simulink model "MP_BearinglessMotor"  (R2024b)
settings: Solver=FixedStepAuto  StartTime=0  StopTime=Tend  FixedStep=Tsim  RelTol=1e-3
values from neighbouring files (symbols this model uses):
  alpha_s = 2*pi/m*ps    (= 5.23598775598)    [setup.m]
  alpha_t = 2*pi/m*p    (= 4.18879020479)    [setup.m]
  Fx_hat = 2/m*Kf    (= 0.6)    [setup.m]
  Fy_hat = 2/m*Kf    (= 0.6)    [setup.m]
  Ke = 0.003    [setup.m]
  p = 4    [setup.m]
  tau_hat = 2/m*Kt    (= 0.00666666666667)    [setup.m]
  Tsim = 1e-8    (= 1e-08)    [setup.m]
  V_DC = 160    [setup.m]
libraries: spsControlledVoltageSourceLib x12, spsIdealSwitchLib x12, spsCurrentMeasurementLib x6, spsMutualInductanceLib x1, spsTriangleGeneratorLib x1, spsVoltageMeasurementLib x1, spsDCVoltageSourceLib x1, spspowerguiLib x1
settings Model: Creator=chiba  LastModifiedBy=tnoguchi
settings SolverCC: AllowMultiTaskInputOutput=on
settings DataIOCC: SaveOutput=off  SaveTime=off
settings OptimizationCC: DefaultParameterBehavior=Inlined  ReuseModelBlockBuffer=off  EnhancedBackFolding=on  PassReuseOutputArgsAs=Individual arguments  ZeroExternalMemoryAtStartup=off  ZeroInternalMemoryAtStartup=off  OptimizeBlockOrder=speed  DifferentSizesBufferReuse=on  EfficientTunableParamExpr=on
settings DebuggingCC: ParameterTunabilityLossMsg=error
settings SFSimCC: MATLABDynamicMemAlloc=off
settings RTWCC: Description=Embedded Coder  SystemTargetFile=ert.tlc  TemplateMakefile=ert_default_tmf  GPUComputeCapability=3.5
settings CodeAppCC: ForceParamTrailComments=on  IgnoreCustomStorageClasses=off  OperatorAnnotations=on  SimulinkDataObjDesc=on  SFDataObjDesc=on  InsertBlockDesc=on
settings ERTTargetCC: TargetLangStandard=C99 (ISO)  ERTCustomFileTemplate=example_file_process.tlc  DynamicArrayContainerType=coder::array

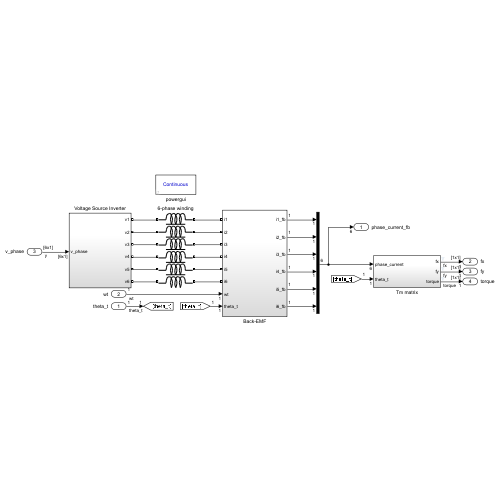
[thumbnail: Simulink's stored preview of the top-level diagram]
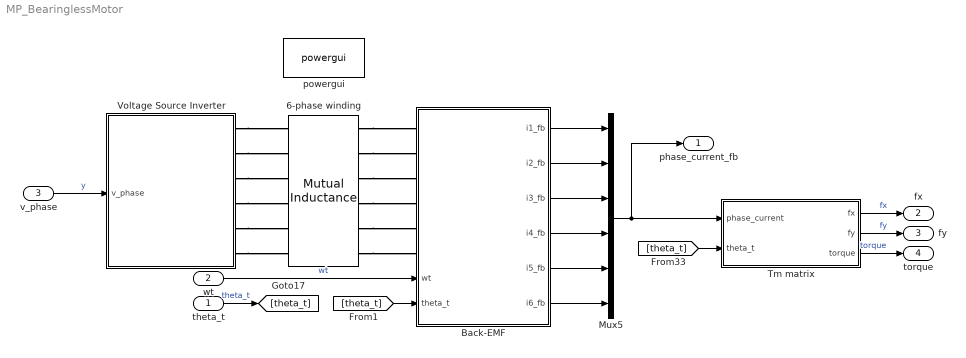
== system MP_BearinglessMotor ==
  theta_t : Inport  OutDataTypeStr=double  PortDimensions=1  SampleTime=0
  wt : Inport  Port=2  OutDataTypeStr=double  PortDimensions=1
  v_phase : Inport  Port=3  OutDataTypeStr=double  PortDimensions=[6 1]  SampleTime=0
  6-phase winding : spsMutualInductanceLib/Mutual Inductance  LConnTagsString=a|b|c|L4|L5|L6  RConnTagsString=A|B|C|R4|R5|R6  TypeOfMutual=Generalized mutual inductance  NumberOfWindings=6  SelfImpedance1=[1.1 1.1e-03]  SelfImpedance2=[ 1.1 1.1e-03]  ThreeWindings=on  SelfImpedance3=[ 1.1 1.1e-03]  MutualImpedance=[1.0 1.0e-03]  InductanceMatrix=Lmat  ResistanceMatrix=Rmat  Measurements=None
      settings: LibrarySourceBlock=sps_lib/Passives/Mutual Inductance
  Back-EMF : Subsystem
      settings: PortSchema="{\"entries\":[{\"content\":{\"sides\":[{\"content\":{\"connectorIds\":[\"LConn1\",\"LConn2\",\"LConn3\",\"LConn4\",\"LConn5\",\"LConn6\",\"In1\",\"In2\"]},\"type\":\"ConnectorPlacement.EquallySpacedRectSide\",\"uuid\":\"749577e6-e43c-48b0-9a92-cb274024c2f1\"},{\"content\":{\"connectorIds\":[\"Out1\",\"Out2\",\"Out3\",\"Out4\",\"Out5\",\"Out6\"],\"side\":\"RIGHT\"},\"type\":\"ConnectorPlacement.EquallySpacedRectSide\",\"uuid\":\"b47f9487-f754-4b9c-a86a-8672228b8979\"},{\"content\":{\"side\":\"TOP\"},\"type\":\"ConnectorPlacement.EquallySpacedRectSide\",\"uuid\":\"ca9d39d3-2f68-4271-a0d3-29a08329b066\"}]},\"type\":\"ConnectorPlacement.EquallySpacedConnector\",\"uuid\":\"24c892f7-b8cb-4be8-a5cc-492343e32fdb\"}],\"packageUris\":[\"http://schema.mathworks.com/mf0/Connector/R2020b\"],\"version\":\"1.0\"}"
  Mux5 : Mux  Inputs=6
  Tm matrix : Subsystem
  Voltage Source Inverter : Subsystem
  powergui : spspowerguiLib/powergui  Priority=1  SimulationMode=Continuous  SampleTime=Tsim  frequency=60  Iterations=50  frequencyindice=0  Pbase=100e6  ErrMax=1e-4  UnitsV=kV  UnitsW=MW  buscounter=0  FunctionMessages=off  echomessages=off  EnableUseOfTLC=off  CurrentSourceSwitches=off  DisableSnubberDevices=off  DisableRonSwitches=off  DisableVfSwitches=off  DisplayEquations=off  AutomaticDiscreteSolvers=off  SolverType=Tustin/Backward Euler (TBE)  Interpol=off  ExternalGateDelay=off  methode=off  Ts=100  x0status=blocks  SPID=on  SwTol=0  HookPort=off  NonlinearTolerance=1e-4  nMaxIteration=100  ContinueOnMaxIteration=off  RestoreLinks=warning  ResistiveCurrentMeasurement=off  Frange=[0:2:500]  Ylog=off  Xlog=on  ShowGrid=off  save=off  variable=ZData  structure=0  ZoomFFT=off  StartTime=0.0  cycles=1  DisplayStyle=1  fundamental=60  FreqAxis=off  MaxFrequency=1000  frequencyindicesteady=1  RmsSteady=1  display=off
  phase_current_fb : Outport  OutDataTypeStr=double  PortDimensions=6  SampleTime=0
  fx : Outport  Port=2  OutDataTypeStr=double  PortDimensions=1  SampleTime=0
  fy : Outport  Port=3  OutDataTypeStr=double  PortDimensions=1  SampleTime=0
  torque : Outport  Port=4  OutDataTypeStr=double  PortDimensions=1  SampleTime=0
  wires:
  Back-EMF/1(i1_fb) -> Mux5/1
  Back-EMF/3(i3_fb) -> Mux5/3
  Back-EMF/2(i2_fb) -> Mux5/2
  Back-EMF/5(i5_fb) -> Mux5/5
  Back-EMF/4(i4_fb) -> Mux5/4
  Back-EMF/6(i6_fb) -> Mux5/6
  [theta_t] -> Tm matrix/2(theta_t)
  Mux5/1 -> Tm matrix/1(phase_current), phase_current_fb/1
  wt/1 -> Back-EMF/1(wt)  "wt"
  [theta_t] -> Back-EMF/2(theta_t)
  theta_t/1 -> [theta_t]  "theta_t"
  v_phase/1 -> Voltage Source Inverter/1(v_phase)  "y"
  Tm matrix/1(fx) -> fx/1  "fx"
  Tm matrix/2(fy) -> fy/1  "fy"
  Tm matrix/3(torque) -> torque/1  "torque"
  connections:
  6-phase winding/RConn1 -- Back-EMF/LConn1
  6-phase winding/RConn2 -- Back-EMF/LConn2
  6-phase winding/RConn3 -- Back-EMF/LConn3
  6-phase winding/RConn4 -- Back-EMF/LConn4
  6-phase winding/RConn5 -- Back-EMF/LConn5
  6-phase winding/RConn6 -- Back-EMF/LConn6
  Voltage Source Inverter/RConn5 -- 6-phase winding/LConn5
  Voltage Source Inverter/RConn6 -- 6-phase winding/LConn6
  Voltage Source Inverter/RConn4 -- 6-phase winding/LConn4
  Voltage Source Inverter/RConn3 -- 6-phase winding/LConn3
  Voltage Source Inverter/RConn2 -- 6-phase winding/LConn2
  Voltage Source Inverter/RConn1 -- 6-phase winding/LConn1

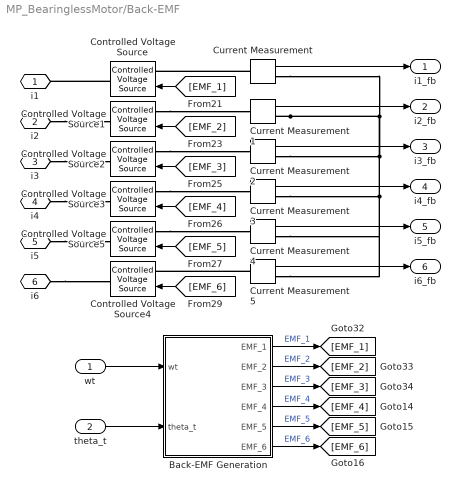
== system MP_BearinglessMotor/Back-EMF ==
  wt : Inport
  theta_t : Inport  Port=2
  Back-EMF Generation : Subsystem
  Controlled Voltage Source{,1..5} (6 alike) : spsControlledVoltageSourceLib/Controlled Voltage Source  Initialize=on  Source_Type=AC  Amplitude=0  Phase=0  Frequency=0  Measurements=None
  Current Measurement{,1..5} (6 alike) : spsCurrentMeasurementLib/Current Measurement  PhasorSimulation=off  OutputType=Complex  PSBequivalent=0
  i1 : PMIOPort  Side=Left
  i2 : PMIOPort  Port=2  Side=Left
  i3 : PMIOPort  Port=3  Side=Left
  i4 : PMIOPort  Port=4  Side=Left
  i5 : PMIOPort  Port=5  Side=Left
  i6 : PMIOPort  Port=6  Side=Left
  i1_fb : Outport
  i2_fb : Outport  Port=2
  i3_fb : Outport  Port=3
  i4_fb : Outport  Port=4
  i5_fb : Outport  Port=5
  i6_fb : Outport  Port=6
  wires:
  Current Measurement2/1 -> i3_fb/1
  Current Measurement4/1 -> i5_fb/1
  Back-EMF Generation/6(EMF_6) -> [EMF_6]  "EMF_6"
  [EMF_4] -> Controlled Voltage Source3/1
  Current Measurement1/1 -> i2_fb/1
  Back-EMF Generation/5(EMF_5) -> [EMF_5]  "EMF_5"
  Current Measurement3/1 -> i4_fb/1
  Back-EMF Generation/2(EMF_2) -> [EMF_2]  "EMF_2"
  [EMF_2] -> Controlled Voltage Source1/1
  [EMF_3] -> Controlled Voltage Source2/1
  [EMF_1] -> Controlled Voltage Source/1
  Current Measurement/1 -> i1_fb/1
  Back-EMF Generation/3(EMF_3) -> [EMF_3]  "EMF_3"
  Back-EMF Generation/4(EMF_4) -> [EMF_4]  "EMF_4"
  [EMF_6] -> Controlled Voltage Source4/1
  Back-EMF Generation/1(EMF_1) -> [EMF_1]  "EMF_1"
  wt/1 -> Back-EMF Generation/1(wt)
  [EMF_5] -> Controlled Voltage Source5/1
  theta_t/1 -> Back-EMF Generation/2(theta_t)
  Current Measurement5/1 -> i6_fb/1
  connections:
  i5/RConn1 -- Controlled Voltage Source5/RConn1
  i3/RConn1 -- Controlled Voltage Source2/RConn1
  Controlled Voltage Source2/LConn1 -- Current Measurement2/LConn1
  i6/RConn1 -- Controlled Voltage Source4/RConn1
  i4/RConn1 -- Controlled Voltage Source3/RConn1
  Controlled Voltage Source1/LConn1 -- Current Measurement1/LConn1
  Current Measurement1/RConn1 -- Current Measurement3/RConn1 -- Current Measurement5/RConn1 -- Current Measurement4/RConn1 -- Current Measurement2/RConn1 -- Current Measurement/RConn1
  Controlled Voltage Source/RConn1 -- i1/RConn1
  Current Measurement/LConn1 -- Controlled Voltage Source/LConn1
  Controlled Voltage Source3/LConn1 -- Current Measurement3/LConn1
  i2/RConn1 -- Controlled Voltage Source1/RConn1
  Controlled Voltage Source5/LConn1 -- Current Measurement4/LConn1
  Current Measurement5/LConn1 -- Controlled Voltage Source4/LConn1

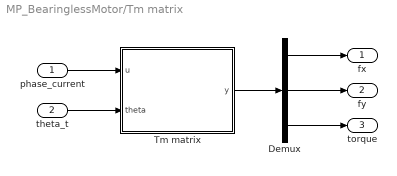
== system MP_BearinglessMotor/Tm matrix ==
  phase_current : Inport
  theta_t : Inport  Port=2
  Demux : Demux  Outputs=3
  Tm matrix : MATLAB Function  TreatAsAtomicUnit=on
  fx : Outport
  fy : Outport  Port=2
  torque : Outport  Port=3
  wires:
  phase_current/1 -> Tm matrix/1(u)
  Tm matrix/1(y) -> Demux/1
  Demux/1 -> fx/1
  Demux/2 -> fy/1
  Demux/3 -> torque/1
  theta_t/1 -> Tm matrix/2(theta)

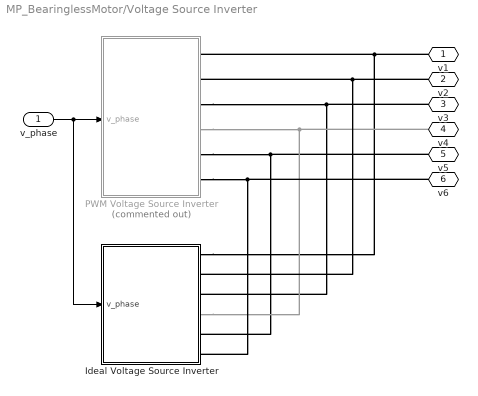
== system MP_BearinglessMotor/Voltage Source Inverter ==
  v_phase : Inport
  Ideal Voltage Source Inverter : Subsystem
  PWM Voltage Source Inverter : Subsystem  Commented=on
  v1 : PMIOPort  Side=Right
  v2 : PMIOPort  Port=2  Side=Right
  v3 : PMIOPort  Port=3  Side=Right
  v4 : PMIOPort  Port=4  Side=Right
  v5 : PMIOPort  Port=5  Side=Right
  v6 : PMIOPort  Port=6  Side=Right
  wires:
  v_phase/1 -> PWM Voltage Source Inverter/1(v_phase), Ideal Voltage Source Inverter/1(v_phase)
  connections:
  Ideal Voltage Source Inverter/RConn5 -- v5/RConn1 -- PWM Voltage Source Inverter/RConn5
  Ideal Voltage Source Inverter/RConn3 -- v3/RConn1 -- PWM Voltage Source Inverter/RConn3
  PWM Voltage Source Inverter/RConn1 -- v1/RConn1 -- Ideal Voltage Source Inverter/RConn1
  PWM Voltage Source Inverter/RConn4 -- v4/RConn1 -- Ideal Voltage Source Inverter/RConn4
  Ideal Voltage Source Inverter/RConn6 -- v6/RConn1 -- PWM Voltage Source Inverter/RConn6
  Ideal Voltage Source Inverter/RConn2 -- v2/RConn1 -- PWM Voltage Source Inverter/RConn2

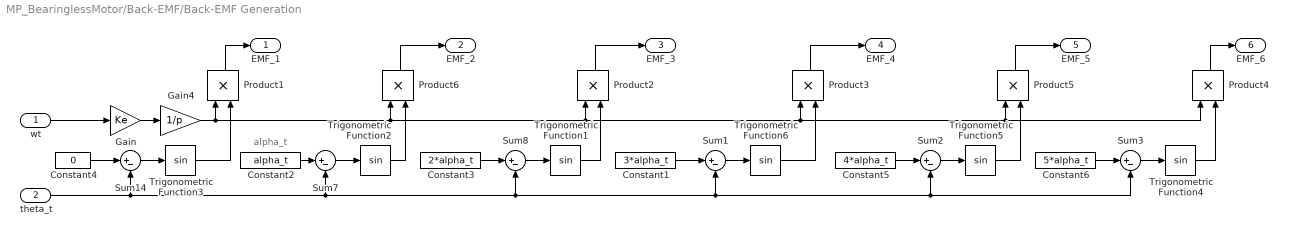
== system MP_BearinglessMotor/Back-EMF/Back-EMF Generation ==
  note: alpha_t
  wt : Inport
  theta_t : Inport  Port=2
  Constant1 : Constant  Value=3*alpha_t
  Constant2 : Constant  Value=alpha_t
  Constant3 : Constant  Value=2*alpha_t
  Constant4 : Constant  Value=0
  Constant5 : Constant  Value=4*alpha_t
  Constant6 : Constant  Value=5*alpha_t
  Gain : Gain  Gain=Ke
  Gain4 : Gain  Gain=1/p
  Product{1..6} (6 alike) : Product
  Sum{1..3,7..8,14} (6 alike) : Sum  Inputs=|+-
  Trigonometric Function{1..6} (6 alike) : Trigonometry
  EMF_1 : Outport
  EMF_2 : Outport  Port=2
  EMF_3 : Outport  Port=3
  EMF_4 : Outport  Port=4
  EMF_5 : Outport  Port=5
  EMF_6 : Outport  Port=6
  wires:
  Constant3/1 -> Sum8/1
  Product3/1 -> EMF_4/1
  Product5/1 -> EMF_5/1
  Product4/1 -> EMF_6/1
  Gain4/1 -> Product6/1, Product2/1, Product5/1, Product4/1, Product3/1, Product1/1
  Sum2/1 -> Trigonometric Function5/1
  Constant1/1 -> Sum1/1
  Constant5/1 -> Sum2/1
  Trigonometric Function5/1 -> Product5/2
  Constant6/1 -> Sum3/1
  Sum1/1 -> Trigonometric Function6/1
  theta_t/1 -> Sum7/2, Sum8/2, Sum2/2, Sum3/2, Sum1/2, Sum14/2
  Trigonometric Function4/1 -> Product4/2
  Trigonometric Function6/1 -> Product3/2
  Sum3/1 -> Trigonometric Function4/1
  Product2/1 -> EMF_3/1
  Product6/1 -> EMF_2/1
  wt/1 -> Gain/1
  Constant2/1 -> Sum7/1
  Product1/1 -> EMF_1/1
  Sum7/1 -> Trigonometric Function2/1
  Trigonometric Function3/1 -> Product1/2
  Sum14/1 -> Trigonometric Function3/1
  Trigonometric Function1/1 -> Product2/2
  Sum8/1 -> Trigonometric Function1/1
  Trigonometric Function2/1 -> Product6/2
  Gain/1 -> Gain4/1
  Constant4/1 -> Sum14/1

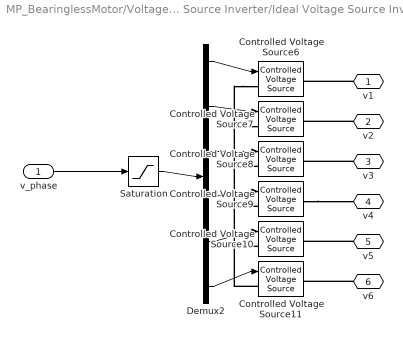
== system MP_BearinglessMotor/Voltage Source Inverter/Ideal Voltage Source Inverter ==
  v_phase : Inport
  Controlled Voltage Source{6..11} (6 alike) : spsControlledVoltageSourceLib/Controlled Voltage Source  Initialize=on  Source_Type=AC  Amplitude=0  Phase=0  Frequency=0  Measurements=None
  Demux2 : Demux  Outputs=6
  Saturation : Saturate  UpperLimit=V_DC/2  LowerLimit=-V_DC/2
  v1 : PMIOPort  Side=Right
  v2 : PMIOPort  Port=2  Side=Right
  v3 : PMIOPort  Port=3  Side=Right
  v4 : PMIOPort  Port=4  Side=Right
  v5 : PMIOPort  Port=5  Side=Right
  v6 : PMIOPort  Port=6  Side=Right
  wires:
  Demux2/1 -> Controlled Voltage Source6/1
  Demux2/4 -> Controlled Voltage Source9/1
  Demux2/5 -> Controlled Voltage Source10/1
  v_phase/1 -> Saturation/1
  Demux2/3 -> Controlled Voltage Source8/1
  Demux2/2 -> Controlled Voltage Source7/1
  Demux2/6 -> Controlled Voltage Source11/1
  Saturation/1 -> Demux2/1
  connections:
  v1/RConn1 -- Controlled Voltage Source6/RConn1
  v3/RConn1 -- Controlled Voltage Source8/RConn1
  v2/RConn1 -- Controlled Voltage Source7/RConn1
  Controlled Voltage Source9/RConn1 -- v4/RConn1
  v5/RConn1 -- Controlled Voltage Source10/RConn1
  v6/RConn1 -- Controlled Voltage Source11/RConn1
  Controlled Voltage Source6/LConn1 -- Controlled Voltage Source8/LConn1 -- Controlled Voltage Source9/LConn1 -- Controlled Voltage Source10/LConn1 -- Controlled Voltage Source11/LConn1 -- Controlled Voltage Source7/LConn1

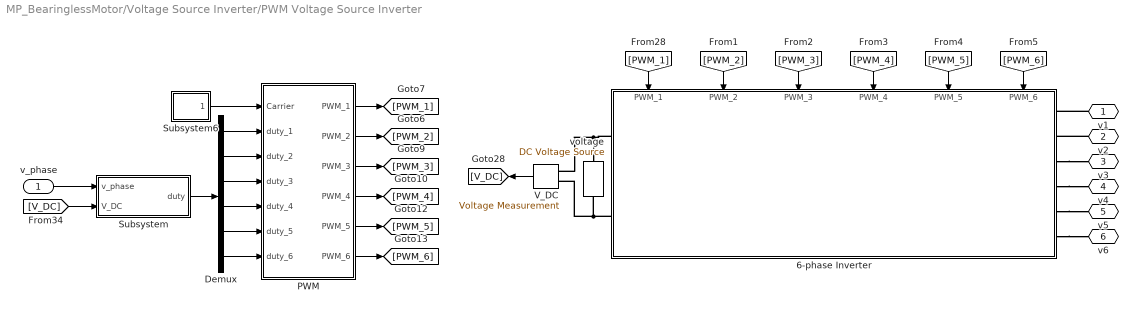
== system MP_BearinglessMotor/Voltage Source Inverter/PWM Voltage Source Inverter ==
  v_phase : Inport
  6-phase Inverter : Subsystem
      settings: PortSchema="{\"entries\":[{\"content\":{\"sides\":[{\"content\":{\"connectorIds\":[\"LConn1\",\"LConn2\"]},\"type\":\"ConnectorPlacement.EquallySpacedRectSide\",\"uuid\":\"ad0dd845-277f-4a71-9690-818fdf3d5926\"},{\"content\":{\"connectorIds\":[\"RConn1\",\"RConn2\",\"RConn3\",\"RConn4\",\"RConn5\",\"RConn6\"],\"side\":\"RIGHT\"},\"type\":\"ConnectorPlacement.EquallySpacedRectSide\",\"uuid\":\"3c53a20e-868e-4f1b-ac43-d8d912ab8c44\"},{\"content\":{\"connectorIds\":[\"In1\",\"In2\",\"In3\",\"In4\",\"In5\",\"In6\"],\"side\":\"TOP\"},\"type\":\"ConnectorPlacement.EquallySpacedRectSide\",\"uuid\":\"cce69e5b-84f2-4b36-9db2-dbef6ebbc603\"},{\"content\":{\"side\":\"BOTTOM\"},\"type\":\"ConnectorPlacement.EquallySpacedRectSide\",\"uuid\":\"85ff7cb9-246d-4834-a807-a84540aa5946\"}]},\"type\":\"ConnectorPlacement.EquallySpacedConnector\",\"uuid\":\"1204721d-d383-4529-bfb2-ba302e152051\"}],\"packageUris\":[\"http://schema.mathworks.com/mf0/Connector/R2020b\"],\"version\":\"1.0\"}"
  Demux : Demux  Outputs=6
  PWM : Subsystem
  Subsystem : Subsystem
  Subsystem6 : Subsystem
  V_DC : spsVoltageMeasurementLib/Voltage Measurement  PhasorSimulation=off  OutputType=Complex  PSBequivalent=0
  voltage : spsDCVoltageSourceLib/DC Voltage Source  Amplitude=V_DC  Measurements=None
  v1 : PMIOPort  Side=Right
  v2 : PMIOPort  Port=2  Side=Right
  v3 : PMIOPort  Port=3  Side=Right
  v4 : PMIOPort  Port=4  Side=Right
  v5 : PMIOPort  Port=5  Side=Right
  v6 : PMIOPort  Port=6  Side=Right
  wires:
  v_phase/1 -> Subsystem/1(v_phase)
  Demux/3 -> PWM/4(duty_3)
  Demux/1 -> PWM/2(duty_1)
  PWM/6(PWM_6) -> [PWM_6]
  [PWM_5] -> 6-phase Inverter/5(PWM_5)
  [PWM_6] -> 6-phase Inverter/6(PWM_6)
  PWM/2(PWM_2) -> [PWM_2]
  [V_DC] -> Subsystem/2(V_DC)
  Demux/4 -> PWM/5(duty_4)
  Demux/2 -> PWM/3(duty_2)
  Subsystem/1(duty) -> Demux/1
  [PWM_4] -> 6-phase Inverter/4(PWM_4)
  PWM/3(PWM_3) -> [PWM_3]
  [PWM_1] -> 6-phase Inverter/1(PWM_1)
  V_DC/1 -> [V_DC]
  PWM/5(PWM_5) -> [PWM_5]
  PWM/1(PWM_1) -> [PWM_1]
  [PWM_3] -> 6-phase Inverter/3(PWM_3)
  PWM/4(PWM_4) -> [PWM_4]
  Demux/6 -> PWM/7(duty_6)
  [PWM_2] -> 6-phase Inverter/2(PWM_2)
  Subsystem6/1(Carrier) -> PWM/1(Carrier)
  Demux/5 -> PWM/6(duty_5)
  connections:
  6-phase Inverter/RConn6 -- v6/RConn1
  v2/RConn1 -- 6-phase Inverter/RConn2
  voltage/LConn1 -- V_DC/LConn2 -- 6-phase Inverter/LConn2
  6-phase Inverter/RConn3 -- v3/RConn1
  6-phase Inverter/RConn4 -- v4/RConn1
  6-phase Inverter/RConn5 -- v5/RConn1
  v1/RConn1 -- 6-phase Inverter/RConn1
  V_DC/LConn1 -- voltage/RConn1 -- 6-phase Inverter/LConn1

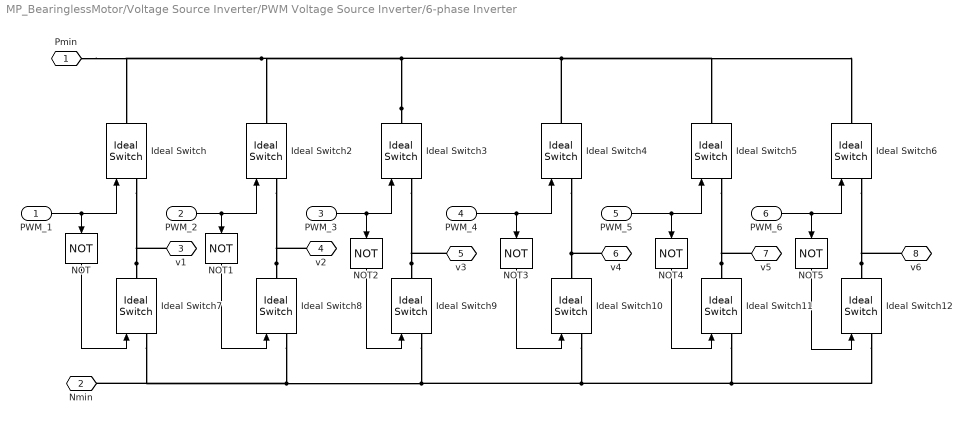
== system MP_BearinglessMotor/Voltage Source Inverter/PWM Voltage Source Inverter/6-phase Inverter ==
  PWM_1 : Inport
  PWM_2 : Inport  Port=2
  PWM_3 : Inport  Port=3
  PWM_4 : Inport  Port=4
  PWM_5 : Inport  Port=5
  PWM_6 : Inport  Port=6
  Ideal Switch{,2..12} (12 alike) : spsIdealSwitchLib/Ideal Switch  Ron=0.00000001  Lon=0  IC=0  Rs=1e5  Cs=inf  Measurements=off
  NOT{,1..5} (6 alike) : Logic  Operator=NOT  IconShape=distinctive  AllPortsSameDT=off  OutDataTypeStr=boolean
  Pmin : PMIOPort  Side=Left
  Nmin : PMIOPort  Port=2  Side=Left
  v1 : PMIOPort  Port=3  Side=Right
  v2 : PMIOPort  Port=4  Side=Right
  v3 : PMIOPort  Port=5  Side=Right
  v4 : PMIOPort  Port=6  Side=Right
  v5 : PMIOPort  Port=7  Side=Right
  v6 : PMIOPort  Port=8  Side=Right
  wires:
  NOT5/1 -> Ideal Switch12/1
  NOT4/1 -> Ideal Switch11/1
  NOT3/1 -> Ideal Switch10/1
  NOT2/1 -> Ideal Switch9/1
  PWM_3/1 -> NOT2/1, Ideal Switch3/1
  NOT1/1 -> Ideal Switch8/1
  NOT/1 -> Ideal Switch7/1
  PWM_6/1 -> Ideal Switch6/1, NOT5/1
  PWM_5/1 -> Ideal Switch5/1, NOT4/1
  PWM_4/1 -> NOT3/1, Ideal Switch4/1
  PWM_2/1 -> NOT1/1, Ideal Switch2/1
  PWM_1/1 -> NOT/1, Ideal Switch/1
  connections:
  Ideal Switch4/LConn1 -- Ideal Switch10/RConn1 -- v4/RConn1
  Ideal Switch12/RConn1 -- Ideal Switch6/LConn1 -- v6/RConn1
  Ideal Switch11/RConn1 -- Ideal Switch5/LConn1 -- v5/RConn1
  Ideal Switch7/RConn1 -- Ideal Switch/LConn1 -- v1/RConn1
  Ideal Switch3/RConn1 -- Ideal Switch4/RConn1 -- Ideal Switch5/RConn1 -- Ideal Switch6/RConn1 -- Ideal Switch2/RConn1 -- Ideal Switch/RConn1 -- Pmin/RConn1
  Ideal Switch8/RConn1 -- Ideal Switch2/LConn1 -- v2/RConn1
  Ideal Switch9/RConn1 -- Ideal Switch3/LConn1 -- v3/RConn1
  Ideal Switch11/LConn1 -- Ideal Switch12/LConn1 -- Ideal Switch10/LConn1 -- Ideal Switch9/LConn1 -- Ideal Switch8/LConn1 -- Ideal Switch7/LConn1 -- Nmin/RConn1

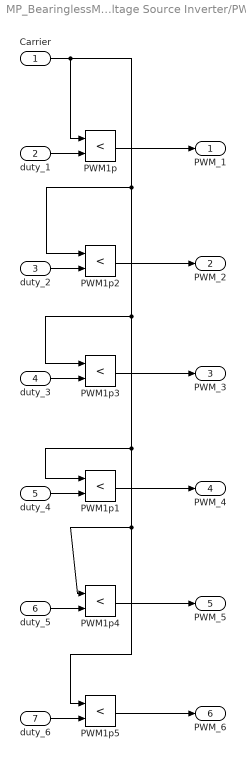
== system MP_BearinglessMotor/Voltage Source Inverter/PWM Voltage Source Inverter/PWM ==
  Carrier : Inport
  duty_1 : Inport  Port=2
  duty_2 : Inport  Port=3
  duty_3 : Inport  Port=4
  duty_4 : Inport  Port=5
  duty_5 : Inport  Port=6
  duty_6 : Inport  Port=7
  PWM1p{,1..5} (6 alike) : RelationalOperator  Operator=<  OutDataTypeStr=boolean  RndMeth=Simplest  InputSameDT=off
  PWM_1 : Outport
  PWM_2 : Outport  Port=2
  PWM_3 : Outport  Port=3
  PWM_4 : Outport  Port=4
  PWM_5 : Outport  Port=5
  PWM_6 : Outport  Port=6
  wires:
  duty_3/1 -> PWM1p3/2
  duty_6/1 -> PWM1p5/2
  duty_5/1 -> PWM1p4/2
  duty_4/1 -> PWM1p1/2
  Carrier/1 -> PWM1p/1, PWM1p5/1, PWM1p4/1, PWM1p1/1, PWM1p3/1, PWM1p2/1
  PWM1p5/1 -> PWM_6/1
  PWM1p/1 -> PWM_1/1
  duty_1/1 -> PWM1p/2
  duty_2/1 -> PWM1p2/2
  PWM1p4/1 -> PWM_5/1
  PWM1p3/1 -> PWM_3/1
  PWM1p2/1 -> PWM_2/1
  PWM1p1/1 -> PWM_4/1

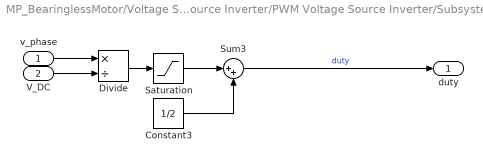
== system MP_BearinglessMotor/Voltage Source Inverter/PWM Voltage Source Inverter/Subsystem ==
  v_phase : Inport
  V_DC : Inport  Port=2
  Constant3 : Constant  Value=1/2
  Divide : Product  Inputs=*/
  Saturation : Saturate
  Sum3 : Sum  Inputs=|++
  duty : Outport
  wires:
  V_DC/1 -> Divide/2
  Sum3/1 -> duty/1  "duty"
  Constant3/1 -> Sum3/2
  v_phase/1 -> Divide/1
  Divide/1 -> Saturation/1
  Saturation/1 -> Sum3/1

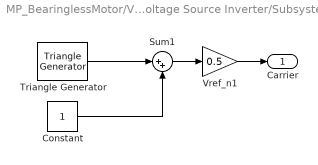
== system MP_BearinglessMotor/Voltage Source Inverter/PWM Voltage Source Inverter/Subsystem6 ==
  Constant : Constant
  Sum1 : Sum  Inputs=|++
  Triangle Generator : spsTriangleGeneratorLib/Triangle Generator  Freq=Fsw  Phase=0  Ts=Tsim
  Vref_n1 : Gain  Gain=0.5
  Carrier : Outport
  wires:
  Vref_n1/1 -> Carrier/1
  Triangle Generator/1 -> Sum1/1
  Constant/1 -> Sum1/2
  Sum1/1 -> Vref_n1/1

== matlab function MP_BearinglessMotor/Tm matrix/Tm matrix ==
  data: u input; y output; theta input; alpha_t parameter; alpha_s parameter; tau_hat parameter; Fx_hat parameter; Fy_hat parameter
function y = fcn(u, theta, alpha_t, alpha_s, tau_hat, Fx_hat, Fy_hat)

Tm = [Fx_hat*cos(theta) Fx_hat*cos(theta-alpha_s) Fx_hat*cos(theta-2*alpha_s) Fx_hat*cos(theta-3*alpha_s) Fx_hat*cos(theta-4*alpha_s) Fx_hat*cos(theta-5*alpha_s);
      Fy_hat*sin(theta) Fy_hat*sin(theta-alpha_s) Fy_hat*sin(theta-2*alpha_s) Fy_hat*sin(theta-3*alpha_s) Fy_hat*sin(theta-4*alpha_s) Fy_hat*sin(theta-5*alpha_s);
      -tau_hat*sin(theta) -tau_hat*sin(theta-alpha_t) -tau_hat*sin(theta-2*alpha_t) -tau_hat*sin(theta-3*alpha_t) -tau_hat*sin(theta-4*alpha_t) -tau_hat*sin(theta-5*alpha_t);];

y = Tm*u;

end
